simulink model "es_4_2018b"  (R2018b)
settings: Solver=VariableStepAuto  StartTime=0.0  StopTime=0.5  RelTol=1e-3
values from neighbouring files (symbols this model uses):
  bit_I = 12    [es4.m]
  bit_PWM = 10    [es4.m]
  C = g/(1+Trm*s)    [es4.m]
  Hi = 1/In    (= 0.0333333333333)    [es4.m]
  Hw = 1/wn    (= 0.00318309886184)    [es4.m]
  In = 30    [es4.m]
  J = 0.0013    [es4.m]
  ki_i = double(-wp_i/abs(B1)*sin(-pi+phiM_i-angle(B1)))    [es4.m]
  ki_s = double(-wp_s/abs(B3)*sin(-pi+phiM_s-angle(B3)))    [es4.m]
  kp_i = double(1/abs(B1)*cos(-pi+phiM_i-angle(B1)))    [es4.m]
  kp_s = double(1/abs(B3)*cos(-pi+phiM_s-angle(B3)))    [es4.m]
  Kt = 0.32    [es4.m]
  ppr_speed = 2000    [es4.m]
  R = 0.32    [es4.m]
  Ti = 1/(1+s*Tsi)    [es4.m]
  Tsi = 0.25e-3    (= 0.00025)    [es4.m]
  Tsw = 1e-3    (= 0.001)    [es4.m]
  Tw = 1/(1+s*Tsw)    [es4.m]
  Vn = 110    [es4.m]
  wn = 3000*pi/30    (= 314.159265359)    [es4.m]
libraries: simulink x2
settings Model: Creator=stefa  LastModifiedBy=Riccardo

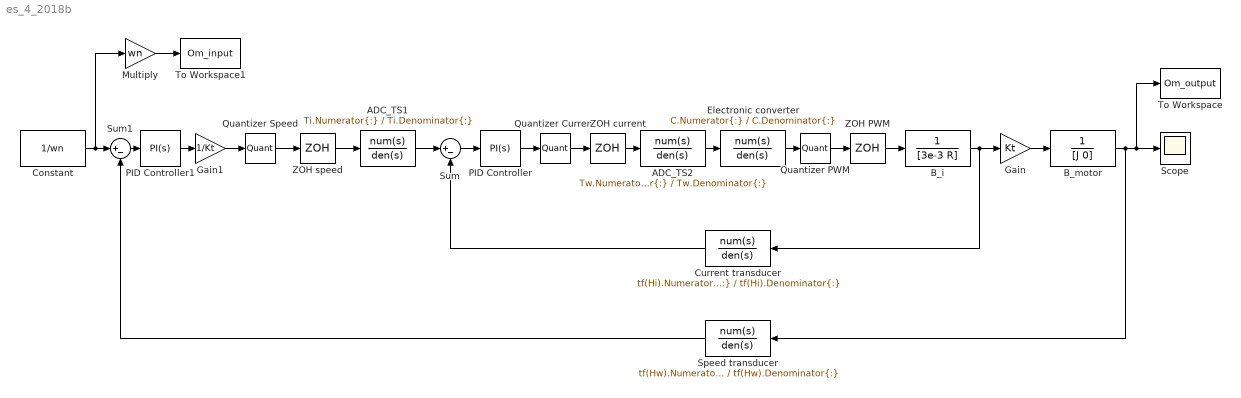
== system es_4_2018b ==
  ADC_TS1 : TransferFcn  Numerator=Ti.Numerator{:}  Denominator=Ti.Denominator{:}
  "ADC_TS2 " : TransferFcn  Numerator=Tw.Numerator{:}  Denominator=Tw.Denominator{:}
  B_i : TransferFcn  Denominator=[3e-3 R]
  B_motor : TransferFcn  Numerator=1  Denominator=[J 0]
  Constant : Constant  Value=1/wn
  Current transducer : TransferFcn  Numerator=tf(Hi).Numerator{:}  Denominator=tf(Hi).Denominator{:}
  Electronic converter : TransferFcn  Numerator=C.Numerator{:}  Denominator=C.Denominator{:}
  Gain : Gain  Gain=Kt
  Gain1 : Gain  Gain=1/Kt
  Multiply : Gain  Gain=wn
  PID Controller : simulink/Continuous/PID Controller  Controller=PI  Form=Parallel  TimeDomain=Continuous-time  SampleTime=-1  IntegratorMethod=Forward Euler  FilterMethod=Forward Euler  ControllerParametersSource=internal  P=kp_i  I=ki_i  D=0  UseFilter=on  N=100  TunerSelectOption=Transfer Function Based (PID Tuner App)  InitialConditionSource=internal  InitialConditionForIntegrator=0  InitialConditionForFilter=0  DifferentiatorICPrevScaledInput=0  ExternalReset=none  TrackingMode=off  Kt=1  LimitOutput=off  UpperSaturationLimit=inf  LowerSaturationLimit=-inf  LinearizeAsGain=on  AntiWindupMode=none  Kb=1  POutMin=[]  POutMax=[]  IOutMin=[]  IOutMax=[]  DOutMin=[]  DOutMax=[]  NOutMin=[]  NOutMax=[]  SumOutMin=[]  SumOutMax=[]  SaturationOutMin=[]  SaturationOutMax=[]  PParamMin=[]  PParamMax=[]  IParamMin=[]  IParamMax=[]  DParamMin=[]  DParamMax=[]  NParamMin=[]  NParamMax=[]  KbParamMin=[]  KbParamMax=[]  KtParamMin=[]  KtParamMax=[]  KbOutMin=[]  KbOutMax=[]  KtOutMin=[]  KtOutMax=[]  IntegratorOutMin=[]  IntegratorOutMax=[]  FilterOutMin=[]  FilterOutMax=[]  SumI1OutMin=[]  SumI1OutMax=[]  SumI2OutMin=[]  SumI2OutMax=[]  SumI3OutMin=[]  SumI3OutMax=[]  SumI4OutMin=[]  SumI4OutMax=[]  SumDOutMin=[]  SumDOutMax=[]  DifferentiatorOutMin=[]  DifferentiatorOutMax=[]  FilterDiffOutCoefMin=[]  FilterDiffOutCoefMax=[]  ReciprocalOutMin=[]  ReciprocalOutMax=[]  SumDenOutMin=[]  SumDenOutMax=[]  SumNumOutMin=[]  SumNumOutMax=[]  DivideOutMin=[]  DivideOutMax=[]  IntegratorContinuousStateAttributes=''  IntegratorStateMustResolveToSignalObject=off  IntegratorRTWStateStorageClass=Auto  FilterContinuousStateAttributes=''  FilterStateMustResolveToSignalObject=off  FilterRTWStateStorageClass=Auto  ParallelPVariant=InternalParameters  IdealPVariant=Disabled  IVariant=InternalParameters  DVariant=Disabled  IntegratorVariant=Continuous  SatVariant=Disabled  AWVariant=Passthrough  PCopyVariant=Disabled  TRVariant=Disabled  FdbkBlocksVariant=Forward  IdealPFdbkVariant=Disabled  SatFdbkVariant=Disabled  DerivativeFilterVariant=Disabled  NVariant=Disabled  NCopyVariant=Disabled_SignalSpec  FilterICVariant=Disabled  IntegratorICVariant=InternalICs  ExternalResetVariant=Disabled  TRSumVariant=Passthrough  SumFdbkVariant=Disabled  SumVariant=Sum_PI
  PID Controller1 : simulink/Continuous/PID Controller  Controller=PI  Form=Parallel  TimeDomain=Continuous-time  SampleTime=-1  IntegratorMethod=Forward Euler  FilterMethod=Forward Euler  ControllerParametersSource=internal  P=kp_s  I=ki_s  D=0  UseFilter=on  N=100  TunerSelectOption=Transfer Function Based (PID Tuner App)  InitialConditionSource=internal  InitialConditionForIntegrator=0  InitialConditionForFilter=0  DifferentiatorICPrevScaledInput=0  ExternalReset=none  TrackingMode=off  Kt=1  LimitOutput=off  UpperSaturationLimit=inf  LowerSaturationLimit=-inf  LinearizeAsGain=on  AntiWindupMode=none  Kb=1  POutMin=[]  POutMax=[]  IOutMin=[]  IOutMax=[]  DOutMin=[]  DOutMax=[]  NOutMin=[]  NOutMax=[]  SumOutMin=[]  SumOutMax=[]  SaturationOutMin=[]  SaturationOutMax=[]  PParamMin=[]  PParamMax=[]  IParamMin=[]  IParamMax=[]  DParamMin=[]  DParamMax=[]  NParamMin=[]  NParamMax=[]  KbParamMin=[]  KbParamMax=[]  KtParamMin=[]  KtParamMax=[]  KbOutMin=[]  KbOutMax=[]  KtOutMin=[]  KtOutMax=[]  IntegratorOutMin=[]  IntegratorOutMax=[]  FilterOutMin=[]  FilterOutMax=[]  SumI1OutMin=[]  SumI1OutMax=[]  SumI2OutMin=[]  SumI2OutMax=[]  SumI3OutMin=[]  SumI3OutMax=[]  SumI4OutMin=[]  SumI4OutMax=[]  SumDOutMin=[]  SumDOutMax=[]  DifferentiatorOutMin=[]  DifferentiatorOutMax=[]  FilterDiffOutCoefMin=[]  FilterDiffOutCoefMax=[]  ReciprocalOutMin=[]  ReciprocalOutMax=[]  SumDenOutMin=[]  SumDenOutMax=[]  SumNumOutMin=[]  SumNumOutMax=[]  DivideOutMin=[]  DivideOutMax=[]  IntegratorContinuousStateAttributes=''  IntegratorStateMustResolveToSignalObject=off  IntegratorRTWStateStorageClass=Auto  FilterContinuousStateAttributes=''  FilterStateMustResolveToSignalObject=off  FilterRTWStateStorageClass=Auto  ParallelPVariant=InternalParameters  IdealPVariant=Disabled  IVariant=InternalParameters  DVariant=Disabled  IntegratorVariant=Continuous  SatVariant=Disabled  AWVariant=Passthrough  PCopyVariant=Disabled  TRVariant=Disabled  FdbkBlocksVariant=Forward  IdealPFdbkVariant=Disabled  SatFdbkVariant=Disabled  DerivativeFilterVariant=Disabled  NVariant=Disabled  NCopyVariant=Disabled_SignalSpec  FilterICVariant=Disabled  IntegratorICVariant=InternalICs  ExternalResetVariant=Disabled  TRSumVariant=Passthrough  SumFdbkVariant=Disabled  SumVariant=Sum_PI
  Quantizer Current : Quantizer  QuantizationInterval=2*In/(2^(bit_I))  LinearizeAsGain=off
  Quantizer PWM : Quantizer  QuantizationInterval=Vn / (2^(bit_PWM))  LinearizeAsGain=off
  "Quantizer Speed " : Quantizer  QuantizationInterval=2*pi/(ppr_speed)  LinearizeAsGain=off
  Scope : Scope
  Speed transducer : TransferFcn  Numerator=tf(Hw).Numerator{:}  Denominator=tf(Hw).Denominator{:}
  Sum : Sum  Inputs=|+-
  Sum1 : Sum  Inputs=|+-
  To Workspace : ToWorkspace  VariableName=Om_output  SaveFormat=Timeseries  SampleTime=-1
  To Workspace1 : ToWorkspace  VariableName=Om_input  SaveFormat=Timeseries  SampleTime=-1
  ZOH PWM : ZeroOrderHold  SampleTime=-1
  ZOH current : ZeroOrderHold  SampleTime=Tsi
  ZOH speed : ZeroOrderHold  SampleTime=Tsw
  wires:
  Electronic converter/1 -> Quantizer PWM/1
  PID Controller/1 -> Quantizer Current/1
  Sum/1 -> PID Controller/1
  B_i/1 -> Gain/1, Current transducer/1
  Current transducer/1 -> Sum/2
  "ADC_TS2 "/1 -> Electronic converter/1
  Gain/1 -> B_motor/1
  B_motor/1 -> Scope/1, To Workspace/1, Speed transducer/1
  Sum1/1 -> PID Controller1/1
  PID Controller1/1 -> Gain1/1
  Gain1/1 -> "Quantizer Speed "/1
  ADC_TS1/1 -> Sum/1
  Speed transducer/1 -> Sum1/2
  Constant/1 -> Multiply/1, Sum1/1
  Quantizer Current/1 -> ZOH current/1
  Quantizer PWM/1 -> ZOH PWM/1
  ZOH speed/1 -> ADC_TS1/1
  ZOH current/1 -> "ADC_TS2 "/1
  ZOH PWM/1 -> B_i/1
  "Quantizer Speed "/1 -> ZOH speed/1
  Multiply/1 -> To Workspace1/1
